simulink model "freq_2"  (R2018b)
settings: Solver=VariableStepAuto  StartTime=0.0  StopTime=60  RelTol=1e-3
values from neighbouring files (symbols this model uses):
  A = [ -3 0; 1 0 ]    [freq2.m]
  B = [ 1; 0 ]    [freq2.m]
  C1 = [ 1 0 ]    [freq2.m]
  C2 = [ 0 1 ]    [freq2.m]
  Ca = [1 0; 0 1]    [freq2.m]
  Da = [0; 0]    [freq2.m]
  h = 0.5    [freq2.m]
  L = [0 1] * inv(Wc) * (phi^2 + p1 * phi + p2 * eye(2))    [freq2.m]
  Lc = ganho_dc/( C*inv( eye(2) - phi_cl )*gama )    [freq2.m]
  xobs = [0.2 0.2]'    [freq2.m]
settings Model: Creator=fredericovaz  LastModifiedBy=fredericovaz

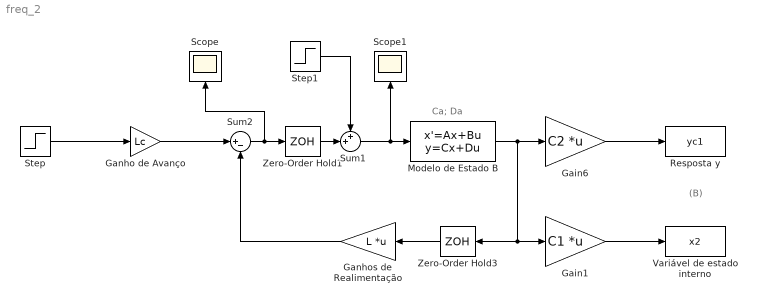
== system freq_2 ==
  note: Ca; Da
  note: (B)
  Gain1 : Gain  Gain=C1  Multiplication=Matrix(K*u) (u vector)
  Gain6 : Gain  Gain=C2  Multiplication=Matrix(K*u) (u vector)
  Ganho de Avanço : Gain  Gain=Lc
  Ganhos de Realimentação : Gain  Gain=L  Multiplication=Matrix(K*u) (u vector)
  Modelo de Estado B : StateSpace  A=A  B=B  C=Ca  D=Da  InitialCondition=xobs
  Resposta y : ToWorkspace  VariableName=yc1  SaveFormat=Structure With Time  SampleTime=-1
  Scope : Scope
  Scope1 : Scope
  Step : Step  Time=10  SampleTime=0
  Step1 : Step  Time=25  Before=0.5  SampleTime=0
  Sum1 : Sum  Inputs=++|
  Sum2 : Sum  Inputs=|+-
  Variável de estado interno : ToWorkspace  VariableName=x2  SaveFormat=Structure With Time  SampleTime=-1
  Zero-Order Hold1 : ZeroOrderHold  SampleTime=h
  Zero-Order Hold3 : ZeroOrderHold  SampleTime=h
  wires:
  Zero-Order Hold3/1 -> Ganhos de Realimentação/1
  Ganhos de Realimentação/1 -> Sum2/2
  Ganho de Avanço/1 -> Sum2/1
  Gain1/1 -> Variável de estado interno/1
  Gain6/1 -> Resposta y/1
  Sum2/1 -> Zero-Order Hold1/1, Scope/1
  Modelo de Estado B/1 -> Zero-Order Hold3/1, Gain1/1, Gain6/1
  Step/1 -> Ganho de Avanço/1
  Zero-Order Hold1/1 -> Sum1/2
  Sum1/1 -> Scope1/1, Modelo de Estado B/1
  Step1/1 -> Sum1/1
